simulink model "sim"  (R2017a)
settings: Solver=FixedStepDiscrete  StartTime=0.0  StopTime=inf  FixedStep=0.001  RelTol=1e-3  EnableMultiTasking=on
undefined symbols (not defined in the file): serial
libraries: simulink x4, instrumentlib x3
settings Model: SimulationMode=accelerator  Creator=VarvaR  LastModifiedBy=tarra
settings OptimizationCC: DefaultParameterBehavior=Inlined  PassReuseOutputArgsAs=Individual arguments  MaxStackSize=64
settings DebuggingCC: ParameterTunabilityLossMsg=error
settings HardwareCC: ProdBitPerPointer=32  ProdBitPerSizeT=32  ProdBitPerPtrDiffT=32  ProdLargestAtomicInteger=Long  ProdLargestAtomicFloat=Double  ProdWordSize=32  ProdHWDeviceType=ARM Compatible->ARM Cortex
settings SFSimCC: MATLABDynamicMemAlloc=off
settings RTWCC: SystemTargetFile=ert.tlc  TemplateMakefile=ert_default_tmf  Description=Embedded Coder  GenerateReport=on  Toolchain=GNU Tools for ARM Embedded Processors  IncludeHyperlinkInReport=on  LaunchReport=on  GenerateTraceInfo=on  GenerateTraceReport=on  GenerateTraceReportSl=on  GenerateTraceReportSf=on  GenerateTraceReportEml=on
settings CodeAppCC: ForceParamTrailComments=on  IgnoreCustomStorageClasses=off  OperatorAnnotations=on  SimulinkDataObjDesc=on  SFDataObjDesc=on  MATLABFcnDesc=on  InsertBlockDesc=on  MATLABSourceComments=on
settings ERTTargetCC: CodeReplacementLibrary=ARM Cortex-M (Optimized)  ERTCustomFileTemplate=example_file_process.tlc

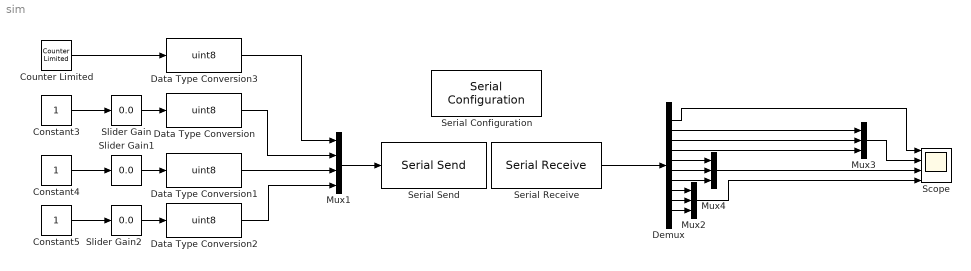
== system sim ==
  Constant3 : Constant  SampleTime=0.1
  Constant4 : Constant  SampleTime=0.1
  Constant5 : Constant  SampleTime=0.1
  Counter Limited : simulink/Sources/Counter Limited  uplimit=10  tsamp=0.1
  Data Type Conversion{,1..3} (4 alike) : DataTypeConversion  OutDataTypeStr=uint8
  Demux : Demux  Outputs=10
  Mux1 : Mux
  Mux2 : Mux  Inputs=3
  Mux3 : Mux  Inputs=3
  Mux4 : Mux  Inputs=3
  Scope : Scope  NumInputPorts=4
  Serial Configuration : instrumentlib/Serial Configuration  Priority=-200000  ComPortMenu=COM6  ComPort=COM6  ObjConstructor=serial('COM6');  BaudRate=500000  DataBits=8  Parity=none  StopBits=1  FlowControl=none  Timeout=10  ByteOrder=LittleEndian
  Serial Receive : instrumentlib/Serial Receive  ComPortMenu=COM6  ComPort=COM6  ObjConstructor=serial('COM6');  Terminator=<none>  DataSize="[1  10]"  DataType=uint16  EnableBlockingMode=on  ActionDataUnavailable=Output last received value  CustomValue=0  SampleTime=0.01
  Serial Send : instrumentlib/Serial Send  ComPortMenu=COM6  ComPort=COM6  ObjConstructor=serial('COM6');  Terminator=<none>  EnableBlockingMode=on
  Slider Gain : simulink/Math Operations/Slider Gain  gain=0.0  low=0  high=100
  Slider Gain1 : simulink/Math Operations/Slider Gain  gain=0.0  low=0  high=100
  Slider Gain2 : simulink/Math Operations/Slider Gain  gain=0.0  low=0  high=100
  wires:
  Serial Receive/1 -> Demux/1
  Demux/1 -> Scope/1
  Demux/2 -> Mux3/1
  Demux/3 -> Mux3/2
  Demux/4 -> Mux3/3
  Demux/5 -> Mux4/1
  Demux/6 -> Mux4/2
  Demux/7 -> Mux4/3
  Mux1/1 -> Serial Send/1
  Data Type Conversion/1 -> Mux1/2
  Data Type Conversion1/1 -> Mux1/3
  Data Type Conversion2/1 -> Mux1/4
  Constant3/1 -> Slider Gain/1
  Slider Gain1/1 -> Data Type Conversion1/1
  Constant4/1 -> Slider Gain1/1
  Counter Limited/1 -> Data Type Conversion3/1
  Constant5/1 -> Slider Gain2/1
  Slider Gain2/1 -> Data Type Conversion2/1
  Slider Gain/1 -> Data Type Conversion/1
  Data Type Conversion3/1 -> Mux1/1
  Demux/8 -> Mux2/1
  Demux/9 -> Mux2/2
  Demux/10 -> Mux2/3
  Mux2/1 -> Scope/4
  Mux4/1 -> Scope/3
  Mux3/1 -> Scope/2
